simulink model "test"  (R2021a)
settings: Solver=ode45  StartTime=0.0  StopTime=1000  FixedStep=0.01  MaxStep=1e-3  RelTol=1e-3
settings Model: Creator=Admin  LastModifiedBy=Admin

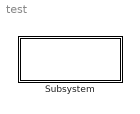
== system test ==
  Subsystem : Subsystem

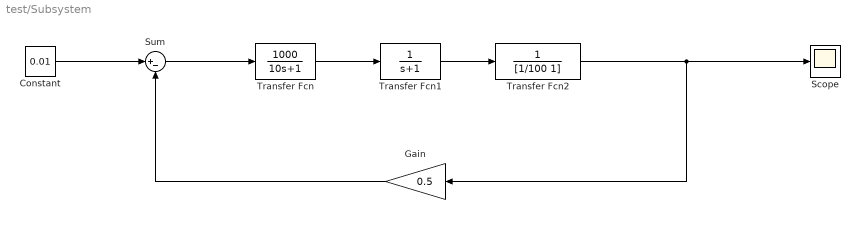
== system test/Subsystem ==
  Constant : Constant  Value=0.01
  Gain : Gain  Gain=0.5
  Scope : Scope
  Sum : Sum  Inputs=|+-
  Transfer Fcn : TransferFcn  Numerator=[1000]  Denominator=[10 1]
  Transfer Fcn1 : TransferFcn  Denominator=[1 1]
  Transfer Fcn2 : TransferFcn  Denominator=[1/100 1]
  wires:
  Transfer Fcn/1 -> Transfer Fcn1/1
  Transfer Fcn1/1 -> Transfer Fcn2/1
  Sum/1 -> Transfer Fcn/1
  Constant/1 -> Sum/1
  Transfer Fcn2/1 -> Gain/1, Scope/1
  Gain/1 -> Sum/2
